simulink model "following_observer"  (R2015a)
settings: Solver=ode45  StartTime=0.0  StopTime=10.0  RelTol=1e-3
values from neighbouring files (symbols this model uses):
  A = [0 1 0 0 ... (first row only)    [following.m]    (also in test1.m = [0 1; test2.m = [0 1 0)
  Av = [0 1 0 0 ... (first row only)    [parameter_variation.m]
  B = [0 ... (first row only)    [following.m]
  Bv = [0 1/M1v 0 0]'    [parameter_variation.m]
  C = [0 0 1 0]    [following.m]    (also in test1.m = [0 1]; test2.m = [1 -1 0)
  H = [-K 1]*inv(M0)*[zeros(4,1);1]    [following.m]
  K = -acker(A,B,p)    [following.m]
  L = -acker(A',C',q)'    [following.m]
  x0 = [-0.5 0 0.5 0]'    [parameter_variation.m]
libraries: simulink x1
settings Model: Creator=shohei  LastModifiedBy=shohei

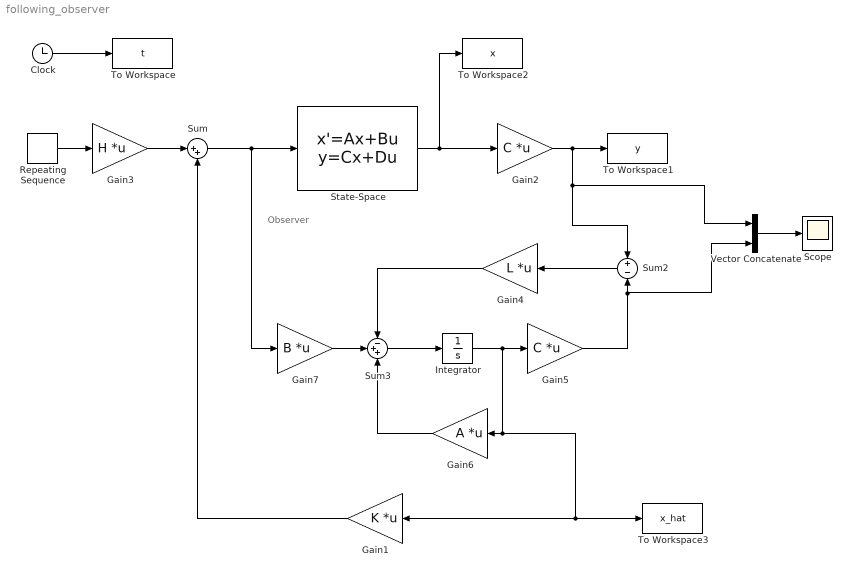
== system following_observer ==
  note: Observer
  Clock : Clock
  Gain1 : Gain  Gain=K  Multiplication=Matrix(K*u)
  Gain2 : Gain  Gain=C  Multiplication=Matrix(K*u)
  Gain3 : Gain  Gain=H  Multiplication=Matrix(K*u)
  Gain4 : Gain  Gain=L  Multiplication=Matrix(K*u)
  Gain5 : Gain  Gain=C  Multiplication=Matrix(K*u)
  Gain6 : Gain  Gain=A  Multiplication=Matrix(K*u)
  Gain7 : Gain  Gain=B  Multiplication=Matrix(K*u)
  Integrator : Integrator
  Repeating Sequence : simulink/Sources/Repeating Sequence  rep_seq_t=[0 2]  rep_seq_y=[0 2]
  Scope : Scope
  State-Space : StateSpace  A=Av  B=Bv  C=eye(4)  D=zeros(4,1)  X0=x0
  Sum : Sum  Inputs=|++
  Sum2 : Sum  Inputs=+|-
  Sum3 : Sum  Inputs=-++
  To Workspace : ToWorkspace  VariableName=t  SampleTime=-1
  To Workspace1 : ToWorkspace  VariableName=y  SampleTime=-1
  To Workspace2 : ToWorkspace  VariableName=x  SampleTime=-1
  To Workspace3 : ToWorkspace  VariableName=x_hat  SampleTime=-1
  Vector Concatenate : Concatenate
  wires:
  State-Space/1 -> To Workspace2/1, Gain2/1
  Clock/1 -> To Workspace/1
  Gain3/1 -> Sum/1
  Repeating Sequence/1 -> Gain3/1
  Gain1/1 -> Sum/2
  Integrator/1 -> To Workspace3/1, Gain1/1, Gain6/1, Gain5/1
  Sum/1 -> Gain7/1, State-Space/1
  Sum2/1 -> Gain4/1
  Gain2/1 -> Vector Concatenate/1, Sum2/1, To Workspace1/1
  Gain5/1 -> Vector Concatenate/2, Sum2/2
  Gain4/1 -> Sum3/1
  Gain6/1 -> Sum3/3
  Sum3/1 -> Integrator/1
  Gain7/1 -> Sum3/2
  Vector Concatenate/1 -> Scope/1
